simulink model "lyskawaLab4_si"  (R2023b)
settings: Solver=VariableStepAuto  StartTime=0.0  StopTime=3  MaxStep=0.05  RelTol=1e-3
values from neighbouring files (symbols this model uses):
  a0 = 6    [lyskawaLab4.m]
  a1 = 2    [lyskawaLab4.m]
  b = 4    [lyskawaLab4.m]
  du = 3    [lyskawaLab4.m]
  t0 = 1.25    [lyskawaLab4.m]
  u0 = 2    [lyskawaLab4.m]
  x0 = 0    [lyskawaLab4.m]
settings Model: Creator=aleklyskawa  LastModifiedBy=aleklyskawa

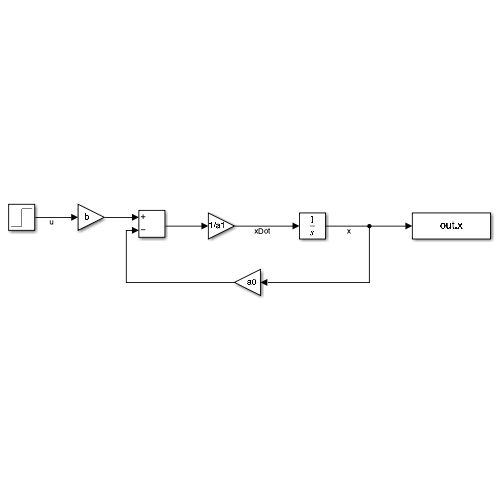
[thumbnail: Simulink's stored preview of the top-level diagram]
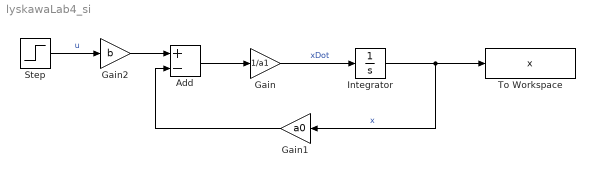
== system lyskawaLab4_si ==
  Add : Sum  Inputs=+-
  Gain : Gain  Gain=1/a1
  Gain1 : Gain  Gain=a0
  Gain2 : Gain  Gain=b
  Integrator : Integrator  InitialCondition=x0
  Step : Step  Time=t0  Before=u0  After=u0 + du  SampleTime=0
  To Workspace : ToWorkspace  VariableName=x  SampleTime=-1
  wires:
  Add/1 -> Gain/1
  Gain/1 -> Integrator/1  "xDot"
  Integrator/1 -> To Workspace/1, Gain1/1  "x"
  Gain1/1 -> Add/2
  Step/1 -> Gain2/1  "u"
  Gain2/1 -> Add/1
